simulink model "Lecture_4_Model1"  (R2021a)
settings: Solver=VariableStepAuto  StartTime=0.0  StopTime=1000  RelTol=1e-3
libraries: fl_lib x11, nesl_utility x6
settings Model: Creator=Admin  LastModifiedBy=Admin

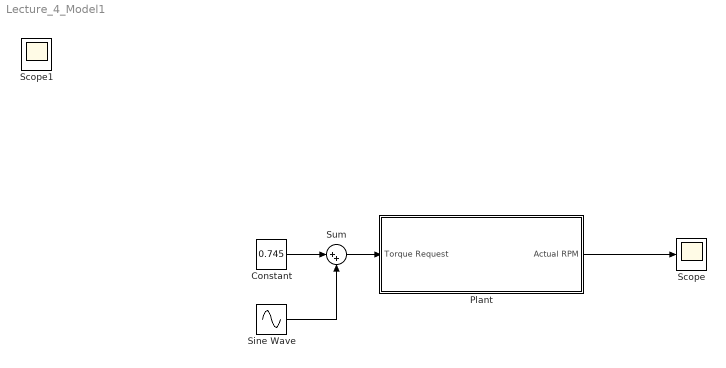
== system Lecture_4_Model1 ==
  Constant : Constant  Value=0.745
  Plant : Subsystem
  Scope : Scope
  Sine Wave : Sin  Amplitude=0.01  Frequency=0.1  SampleTime=0
  Sum : Sum  Inputs=|++
  Scope1 : Scope
  wires:
  Plant/1(Actual RPM) -> Scope/1
  Constant/1 -> Sum/1
  Sum/1 -> Plant/1(Torque Request)
  Sine Wave/1 -> Sum/2

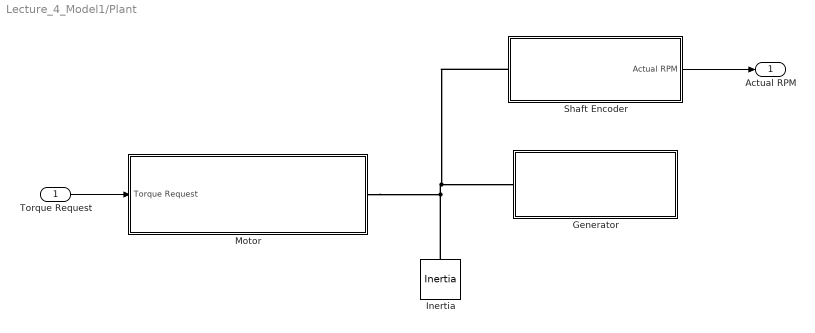
== system Lecture_4_Model1/Plant ==
  Torque Request : Inport
  "Generator " : Subsystem
  Inertia : fl_lib/Mechanical/Rotational Elements/Inertia  inertia=1.041e-4 kg*m^2  num_ports=foundation.enum.numPorts2.one  w_specify=off  w_priority=High  w=0 rad/s  w_nominal_specify=off  w_nominal_unit=rad/s  w_nominal_value=1  t_specify=off  t_priority=None  t=0 N*m  t_nominal_specify=off  t_nominal_unit=N*m  t_nominal_value=1
  "Motor " : Subsystem
  Shaft Encoder : Subsystem
  Actual RPM : Outport
  wires:
  Torque Request/1 -> "Motor "/1(Torque Request)
  Shaft Encoder/1(Actual RPM) -> Actual RPM/1
  connections:
  "Motor "/RConn1 -- Inertia/LConn1 -- "Generator "/LConn1 -- Shaft Encoder/LConn1

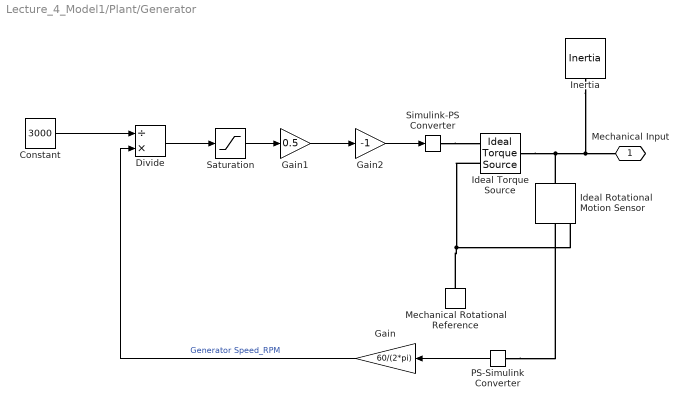
== system Lecture_4_Model1/Plant/Generator  ==
  Constant : Constant  Value=3000
  Divide : Product  Inputs=/*
  Gain : Gain  Gain=60/(2*pi)
  Gain1 : Gain  Gain=0.5
  Gain2 : Gain  Gain=-1
  Ideal Rotational Motion Sensor : fl_lib/Mechanical/Mechanical Sensors/Ideal Rotational Motion Sensor  wrap_angle=simscape.enum.onoff.off  offset=0 rad
  Ideal Torque Source : fl_lib/Mechanical/Mechanical Sources/Ideal Torque Source
  Inertia : fl_lib/Mechanical/Rotational Elements/Inertia  inertia=1e-3 kg*m^2  num_ports=foundation.enum.numPorts2.one  w_specify=on  w_priority=High  w=0 rpm  w_nominal_specify=off  w_nominal_unit=rad/s  w_nominal_value=1  t_specify=off  t_priority=None  t=0 N*m  t_nominal_specify=off  t_nominal_unit=N*m  t_nominal_value=1
  Mechanical Rotational Reference : fl_lib/Mechanical/Rotational Elements/Mechanical Rotational Reference
  PS-Simulink Converter : nesl_utility/PS-Simulink Converter  PhysicalDomain=network_engine_domain  SubClassName=ps_output  LeftPortType=input  RightPortType=output  PseudoPeriodic=off  Frequencies=[]  Unit=inherit  AffineConversion=off
      settings: SourceProductBaseCode=PW,SS
  Saturation : Saturate  UpperLimit=1  LowerLimit=0
  Simulink-PS Converter : nesl_utility/Simulink-PS Converter  PhysicalDomain=network_engine_domain  SubClassName=ps_input  LeftPortType=input  RightPortType=output  PseudoPeriodic=off  Frequencies=[]  NoiseDistribution=none  NoiseParameters=[]  Unit=1  AffineConversion=off  FilteringAndDerivatives=provide  SimscapeFilterOrder=1  InputFilterTimeConstant=0.001  UdotUserProvided=0
      settings: SourceProductBaseCode=PW,SS
  Mechanical Input : PMIOPort  Side=Left
  wires:
  PS-Simulink Converter/1 -> Gain/1
  Constant/1 -> Divide/1
  Gain/1 -> Divide/2  "Generator Speed_RPM"
  Divide/1 -> Saturation/1
  Saturation/1 -> Gain1/1
  Gain1/1 -> Gain2/1
  Gain2/1 -> Simulink-PS Converter/1
  connections:
  Ideal Torque Source/LConn1 -- Mechanical Input/RConn1 -- Inertia/LConn1 -- Ideal Rotational Motion Sensor/LConn1
  Ideal Torque Source/RConn2 -- Mechanical Rotational Reference/LConn1 -- Ideal Rotational Motion Sensor/RConn1
  PS-Simulink Converter/LConn1 -- Ideal Rotational Motion Sensor/RConn2
  Simulink-PS Converter/RConn1 -- Ideal Torque Source/RConn1

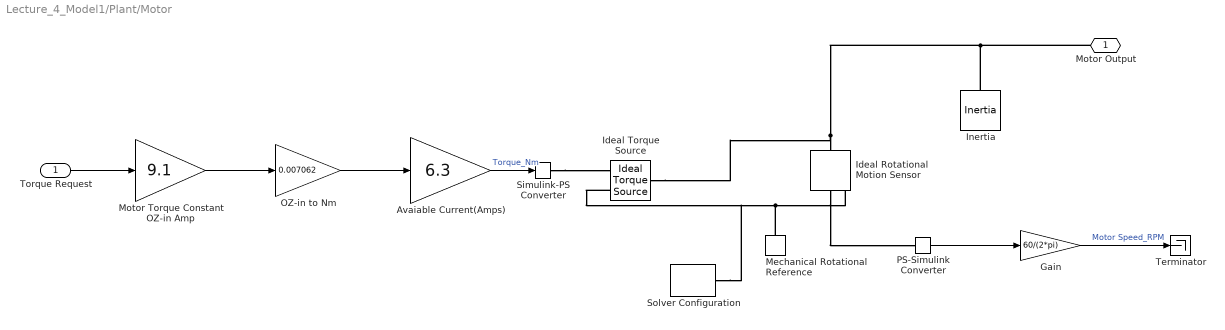
== system Lecture_4_Model1/Plant/Motor  ==
  Torque Request : Inport
  Avaiable Current(Amps) : Gain  Gain=6.3
  Gain : Gain  Gain=60/(2*pi)
  Ideal Rotational Motion Sensor : fl_lib/Mechanical/Mechanical Sensors/Ideal Rotational Motion Sensor  wrap_angle=simscape.enum.onoff.off  offset=0 deg
  Ideal Torque Source : fl_lib/Mechanical/Mechanical Sources/Ideal Torque Source
  Inertia : fl_lib/Mechanical/Rotational Elements/Inertia  inertia=1e-3 kg*m^2  num_ports=foundation.enum.numPorts2.one  w_specify=on  w_priority=High  w=0 rpm  w_nominal_specify=off  w_nominal_unit=rad/s  w_nominal_value=1  t_specify=off  t_priority=None  t=0 N*m  t_nominal_specify=off  t_nominal_unit=N*m  t_nominal_value=1
  Mechanical Rotational Reference : fl_lib/Mechanical/Rotational Elements/Mechanical Rotational Reference
  Motor Torque Constant OZ-in Amp : Gain  Gain=9.1
  OZ-in to Nm : Gain  Gain=0.007062
  PS-Simulink Converter : nesl_utility/PS-Simulink Converter  PhysicalDomain=network_engine_domain  SubClassName=ps_output  LeftPortType=input  RightPortType=output  PseudoPeriodic=off  Frequencies=[]  Unit=inherit  AffineConversion=off
      settings: SourceProductBaseCode=PW,SS
  Simulink-PS Converter : nesl_utility/Simulink-PS Converter  PhysicalDomain=network_engine_domain  SubClassName=ps_input  LeftPortType=input  RightPortType=output  PseudoPeriodic=off  Frequencies=[]  NoiseDistribution=none  NoiseParameters=[]  Unit=1  AffineConversion=off  FilteringAndDerivatives=provide  SimscapeFilterOrder=1  InputFilterTimeConstant=0.001  UdotUserProvided=0
      settings: SourceProductBaseCode=PW,SS
  Solver Configuration : nesl_utility/Solver Configuration  PhysicalDomain=network_engine_domain  SubClassName=solver  LeftPortType=input  RightPortType=generic  Tones=[]  Harmonics=[]  SimulateNoise=off  Profile=off  UseLocalSampling=off  EnableSwitchedLinearOptims=on  FrequencyDomain=off  UseCCode=off  RelTol=0.001  AbsTol=1e-06  MinStep=1e-09  ToWorkspace=off  RevertToSquareIcSolve=off  NumHomotopyIterations=100  PhasorMode=off  PhasorModeNumHarmonics=1  DoDC=off  ResidualTolerance=1e-09  UseLocalSolver=off  LocalSolverChoice=NE_BACKWARD_EULER_ADVANCER  LocalSolverSampleTime=0.001  DoFixedCost=off  MaxNonlinIter=3  MaxModeIter=2  ComputeImpulses=off  ImpulseIterations=2  LinearAlgebra=auto  EquationFormulation=NE_TIME_EF  DelaysMemoryBudget=1024  AutomaticFiltering=on  FilteringTimeConstant=0.001  PartitionStorageMethod=AS_NEEDED  PartitionMemoryBudget=1024  PartitionMethod=ROBUST
      settings: SourceProductBaseCode=PW,SS
  Terminator : Terminator
  Motor Output : PMIOPort  Side=Right
  wires:
  Motor Torque Constant OZ-in Amp/1 -> OZ-in to Nm/1
  OZ-in to Nm/1 -> Avaiable Current(Amps)/1
  Torque Request/1 -> Motor Torque Constant OZ-in Amp/1
  Avaiable Current(Amps)/1 -> Simulink-PS Converter/1  "Torque_Nm"
  PS-Simulink Converter/1 -> Gain/1
  Gain/1 -> Terminator/1  "Motor Speed_RPM"
  connections:
  Motor Output/RConn1 -- Inertia/LConn1 -- Ideal Torque Source/LConn1 -- Ideal Rotational Motion Sensor/LConn1
  Mechanical Rotational Reference/LConn1 -- Solver Configuration/RConn1 -- Ideal Torque Source/RConn2 -- Ideal Rotational Motion Sensor/RConn1
  Ideal Rotational Motion Sensor/RConn2 -- PS-Simulink Converter/LConn1
  Simulink-PS Converter/RConn1 -- Ideal Torque Source/RConn1

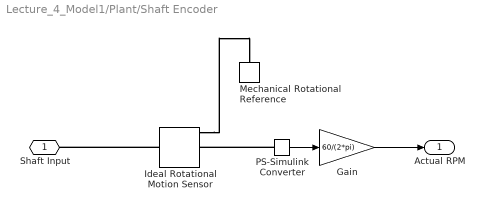
== system Lecture_4_Model1/Plant/Shaft Encoder ==
  Gain : Gain  Gain=60/(2*pi)
  Ideal Rotational Motion Sensor : fl_lib/Mechanical/Mechanical Sensors/Ideal Rotational Motion Sensor  wrap_angle=simscape.enum.onoff.off  offset=0 rad
  Mechanical Rotational Reference : fl_lib/Mechanical/Rotational Elements/Mechanical Rotational Reference
  PS-Simulink Converter : nesl_utility/PS-Simulink Converter  PhysicalDomain=network_engine_domain  SubClassName=ps_output  LeftPortType=input  RightPortType=output  PseudoPeriodic=off  Frequencies=[]  Unit=inherit  AffineConversion=off
      settings: SourceProductBaseCode=PW,SS
  Shaft Input : PMIOPort  Side=Left
  Actual RPM : Outport
  wires:
  PS-Simulink Converter/1 -> Gain/1
  Gain/1 -> Actual RPM/1
  connections:
  Ideal Rotational Motion Sensor/LConn1 -- Shaft Input/RConn1
  Ideal Rotational Motion Sensor/RConn1 -- Mechanical Rotational Reference/LConn1
  PS-Simulink Converter/LConn1 -- Ideal Rotational Motion Sensor/RConn2
